simulink model "linefault"  (Simulink 8.5)
settings: Solver=ode15s  SolverMode=SingleTasking  StartTime=0.0  StopTime=0.1  RelTol=1e-3  AbsTol=1e-6
libraries: powerlib x43, powerlib_extras x1
settings Model: Creator=Dr. Lotfifard  LastModifiedBy=PC  ExtModeTrigMode=oneshot  ExtModeArmWhenConnect=off
settings SolverCC: ZeroCrossAlgorithm=Adaptive
settings DataIOCC: LimitDataPoints=off
settings OptimizationCC: BlockReduction=off  BooleanDataType=off
settings DebuggingCC: SaveWithParameterizedLinksMsg=none  SignalResolutionControl=TryResolveAllWithWarning  MultiTaskDSMMsg=warning  MultiTaskCondExecSysMsg=none  FcnCallInpInsideContextMsg=UseLocalSettings
settings HardwareCC: TargetUnknown=on

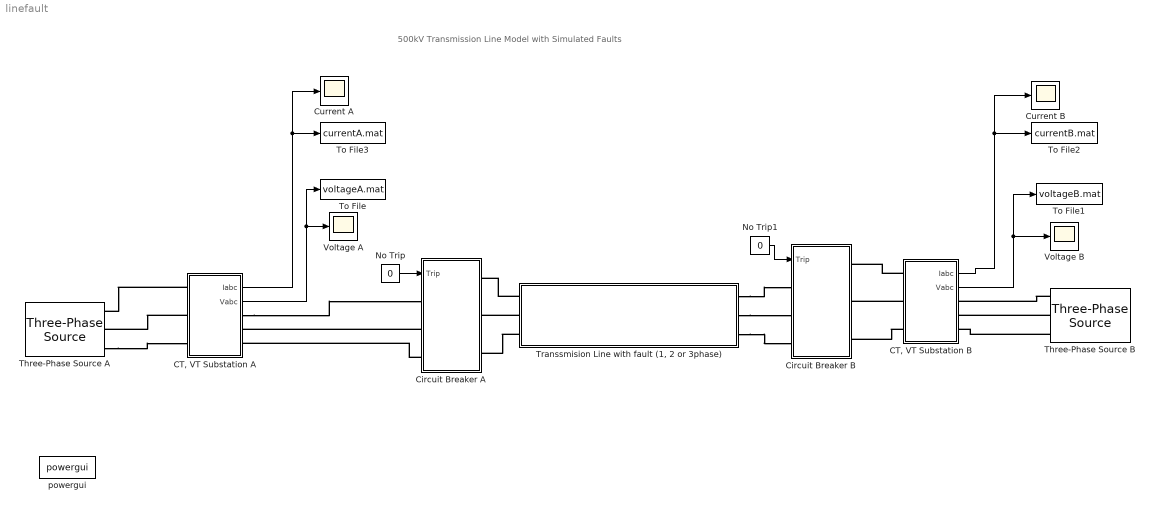
== system linefault ==
  note: 500kV Transmission Line Model with Simulated Faults
  "CT, VT Substation A" : Subsystem  mask{VT=1, CT=1}
      mask prompts: VT "VT ratio"; CT "CT ratio"
  "CT, VT Substation B" : Subsystem  mask{VT=1, CT=1}
      mask prompts: VT "VT ratio"; CT "CT ratio"
  Circuit Breaker A : Subsystem
  Circuit Breaker B : Subsystem
  Current A : Scope
      settings: TickLabels=on  YMin=-8000  YMax=9000
  Current B : Scope
      settings: TickLabels=on
  No Trip : Constant  Value=0
  No Trip1 : Constant  Value=0
  Three-Phase Source A : powerlib/Electrical Sources/Three-Phase Source  Voltage=500000/sqrt(3)*sqrt(2)  PhaseAngle=0  Frequency=60  InternalConnection=Yg  SpecifyImpedance=off  Resistance=0.724  Inductance=19.2e-3  ShortCircuitLevel=100e6  BaseVoltage=25e3  XRratio=7  BusType=swing  Pref=0  Qref=0  Qmin=-inf  Qmax=inf
  Three-Phase Source B : powerlib/Electrical Sources/Three-Phase Source  Voltage=1.05*500000/sqrt(3)*sqrt(2)  PhaseAngle=10  Frequency=60  InternalConnection=Yg  SpecifyImpedance=off  Resistance=0.724  Inductance=19.2e-3  ShortCircuitLevel=100e6  BaseVoltage=25e3  XRratio=7  BusType=swing  Pref=0  Qref=0  Qmin=-inf  Qmax=inf
  To File : ToFile  Filename=voltageA.mat
  To File1 : ToFile  Filename=voltageB.mat
  To File2 : ToFile  Filename=currentB.mat
  To File3 : ToFile  Filename=currentA.mat
  "Transsmision Line with fault (1, 2 or 3phase)" : Subsystem  mask(Teansmission line with fault){ff=60, rr=[0.025485 0.57504], ll=[1.5760e-3 4.5291e-3], cc=[19.1e-9 11.2e-9], length=200, faultLocation=0.1, faultType='A-B', faultR=1, faultTime=[0.034 0.1 0.2 0.5 1]}
      mask prompts: ff "Frequency used for R L C specification (Hz)"; rr "Resistance per unit length (Ohm/km) [R1 R0]"; ll "Inductance per unit length (H/km) [L1 L0]"; cc "Capacitance per unit length (F/km) [C1 C0]"; length "Line length (km)"; faultLocation "Fault location (p.u.) <0,1>"; faultType "Fault Type"; faultR "Fault Resistance per Phase (Ohm)"; faultTime "Fault time sequence (s) [C O C O C]"
      mask TypeOptions faultType: 'A-G' | 'A-B' | 'A-B-G' | 'A-B-C' | 'A-B-C-G'
  Voltage A : Scope
      settings: TickLabels=on
  Voltage B : Scope
      settings: TickLabels=on
  powergui : powerlib/powergui  SimulationMode=Continuous  SolverType=Tustin/Backward Euler (TBE)  SampleTime=0  frequency=60  SPID=off  DisableSnubberDevices=off  DisableRonSwitches=off  DisableVfSwitches=off  SwTol=0  DisplayEquations=off  Interpol=off  methode=off  Ts=0  FunctionMessages=off  echomessages=off  HookPort=off  EnableUseOfTLC=off  x0status=blocks  frequencyindice=60  Pbase=100e6  ErrMax=1e-4  Iterations=50  UnitsV=kV  UnitsW=MW  buscounter=0  RestoreLinks=warning  ResistiveCurrentMeasurement=off  Frange=[0:2:500]  Ylog=off  Xlog=on  ShowGrid=off  save=off  variable=ZData  structure=0  ZoomFFT=on  StartTime=0.0  cycles=1  DisplayStyle=1  fundamental=60  FreqAxis=off  MaxFrequency=1000  frequencyindicesteady=1  RmsSteady=1  display=off
  wires:
  No Trip/1 -> Circuit Breaker A/1(Trip)
  "CT, VT Substation A"/2(Vabc) -> Voltage A/1, To File/1
  No Trip1/1 -> Circuit Breaker B/1(Trip)
  "CT, VT Substation B"/1(Iabc) -> To File2/1, Current B/1
  "CT, VT Substation B"/2(Vabc) -> Voltage B/1, To File1/1
  "CT, VT Substation A"/1(Iabc) -> To File3/1, Current A/1
  connections:
  "CT, VT Substation A"/LConn1 -- Three-Phase Source A/RConn1
  Circuit Breaker A/LConn3 -- "CT, VT Substation A"/RConn3
  "CT, VT Substation B"/LConn2 -- Circuit Breaker B/RConn2
  "CT, VT Substation B"/LConn1 -- Circuit Breaker B/RConn1
  "CT, VT Substation B"/LConn3 -- Circuit Breaker B/RConn3
  Three-Phase Source B/RConn2 -- "CT, VT Substation B"/RConn2
  Three-Phase Source B/RConn1 -- "CT, VT Substation B"/RConn1
  Three-Phase Source B/RConn3 -- "CT, VT Substation B"/RConn3
  "Transsmision Line with fault (1, 2 or 3phase)"/LConn3 -- Circuit Breaker A/RConn3
  "Transsmision Line with fault (1, 2 or 3phase)"/LConn2 -- Circuit Breaker A/RConn2
  "Transsmision Line with fault (1, 2 or 3phase)"/LConn1 -- Circuit Breaker A/RConn1
  "Transsmision Line with fault (1, 2 or 3phase)"/RConn1 -- Circuit Breaker B/LConn1
  "Transsmision Line with fault (1, 2 or 3phase)"/RConn2 -- Circuit Breaker B/LConn2
  "Transsmision Line with fault (1, 2 or 3phase)"/RConn3 -- Circuit Breaker B/LConn3
  Three-Phase Source A/RConn3 -- "CT, VT Substation A"/LConn3
  "CT, VT Substation A"/LConn2 -- Three-Phase Source A/RConn2
  "CT, VT Substation A"/RConn1 -- Circuit Breaker A/LConn1
  Circuit Breaker A/LConn2 -- "CT, VT Substation A"/RConn2

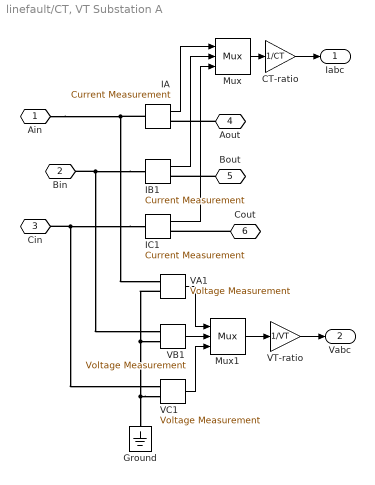
== system linefault/CT, VT Substation A ==
  CT-ratio : Gain  Gain=1/CT  SaturateOnIntegerOverflow=on  OutDataTypeStr=Inherit: Same as input  ParamDataTypeStr=Inherit: Same as input
  Ground : powerlib/Elements/Ground  LConnTagsString=a
  IA : powerlib/Measurements/Current Measurement  PhasorSimulation=off  OutputType=Complex  PSBequivalent=0
  IB1 : powerlib/Measurements/Current Measurement  PhasorSimulation=off  OutputType=Complex  PSBequivalent=0
  IC1 : powerlib/Measurements/Current Measurement  PhasorSimulation=off  OutputType=Complex  PSBequivalent=0
  Mux : Mux  Inputs=3
  Mux1 : Mux  Inputs=3
  VA1 : powerlib/Measurements/Voltage Measurement  PhasorSimulation=off  OutputType=Complex  PSBequivalent=0
  VB1 : powerlib/Measurements/Voltage Measurement  PhasorSimulation=off  OutputType=Complex  PSBequivalent=0
  VC1 : powerlib/Measurements/Voltage Measurement  PhasorSimulation=off  OutputType=Complex  PSBequivalent=0
  VT-ratio : Gain  Gain=1/VT  SaturateOnIntegerOverflow=on  OutDataTypeStr=Inherit: Same as input  ParamDataTypeStr=Inherit: Same as input
  Ain : PMIOPort  Port=1  Side=Left
  Bin : PMIOPort  Port=2  Side=Left
  Cin : PMIOPort  Port=3  Side=Left
  Aout : PMIOPort  Port=4  Side=Right
  Bout : PMIOPort  Port=5  Side=Right
  Cout : PMIOPort  Port=6  Side=Right
  Iabc : Outport
  Vabc : Outport  Port=2
  wires:
  Mux/1 -> CT-ratio/1
  Mux1/1 -> VT-ratio/1
  IA/1 -> Mux/1
  IB1/1 -> Mux/2
  IC1/1 -> Mux/3
  VC1/1 -> Mux1/3
  VB1/1 -> Mux1/2
  VA1/1 -> Mux1/1
  CT-ratio/1 -> Iabc/1
  VT-ratio/1 -> Vabc/1
  connections:
  VC1/LConn2 -- Ground/LConn1 -- VB1/LConn2 -- VA1/LConn2
  Ain/RConn1 -- IA/LConn1 -- VA1/LConn1
  IB1/LConn1 -- Bin/RConn1 -- VB1/LConn1
  IC1/LConn1 -- Cin/RConn1 -- VC1/LConn1
  Cout/RConn1 -- IC1/RConn1
  Aout/RConn1 -- IA/RConn1
  Bout/RConn1 -- IB1/RConn1

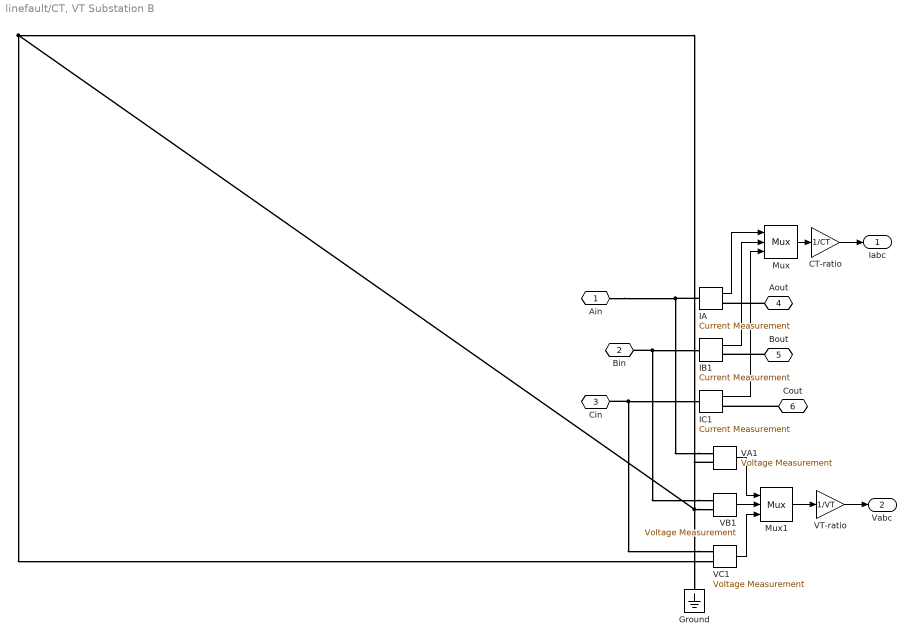
== system linefault/CT, VT Substation B ==
  CT-ratio : Gain  Gain=1/CT  SaturateOnIntegerOverflow=on  OutDataTypeStr=Inherit: Same as input  ParamDataTypeStr=Inherit: Same as input
  Ground : powerlib/Elements/Ground  LConnTagsString=a
  IA : powerlib/Measurements/Current Measurement  PhasorSimulation=off  OutputType=Complex  PSBequivalent=0
  IB1 : powerlib/Measurements/Current Measurement  PhasorSimulation=off  OutputType=Complex  PSBequivalent=0
  IC1 : powerlib/Measurements/Current Measurement  PhasorSimulation=off  OutputType=Complex  PSBequivalent=0
  Mux : Mux  Inputs=3
  Mux1 : Mux  Inputs=3
  VA1 : powerlib/Measurements/Voltage Measurement  PhasorSimulation=off  OutputType=Complex  PSBequivalent=0
  VB1 : powerlib/Measurements/Voltage Measurement  PhasorSimulation=off  OutputType=Complex  PSBequivalent=0
  VC1 : powerlib/Measurements/Voltage Measurement  PhasorSimulation=off  OutputType=Complex  PSBequivalent=0
  VT-ratio : Gain  Gain=1/VT  SaturateOnIntegerOverflow=on  OutDataTypeStr=Inherit: Same as input  ParamDataTypeStr=Inherit: Same as input
  Ain : PMIOPort  Port=1  Side=Left
  Bin : PMIOPort  Port=2  Side=Left
  Cin : PMIOPort  Port=3  Side=Left
  Aout : PMIOPort  Port=4  Side=Right
  Bout : PMIOPort  Port=5  Side=Right
  Cout : PMIOPort  Port=6  Side=Right
  Iabc : Outport
  Vabc : Outport  Port=2
  wires:
  Mux/1 -> CT-ratio/1
  Mux1/1 -> VT-ratio/1
  IA/1 -> Mux/1
  IB1/1 -> Mux/2
  IC1/1 -> Mux/3
  VC1/1 -> Mux1/3
  VB1/1 -> Mux1/2
  VA1/1 -> Mux1/1
  CT-ratio/1 -> Iabc/1
  VT-ratio/1 -> Vabc/1
  connections:
  VB1/LConn2 -- VA1/LConn2 -- VC1/LConn2 -- Ground/LConn1
  VA1/LConn1 -- Ain/RConn1 -- IA/LConn1
  VB1/LConn1 -- IB1/LConn1 -- Bin/RConn1
  VC1/LConn1 -- IC1/LConn1 -- Cin/RConn1
  Cout/RConn1 -- IC1/RConn1
  Aout/RConn1 -- IA/RConn1
  Bout/RConn1 -- IB1/RConn1

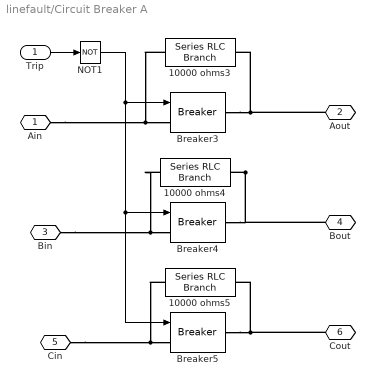
== system linefault/Circuit Breaker A ==
  Trip : Inport
  10000 ohms3 : powerlib/Elements/Series RLC Branch  LConnTagsString=__new0  RConnTagsString=__new0  BranchType=R  Resistance=10000  Inductance=1e-3  SetiL0=off  InitialCurrent=0  Capacitance=1e-6  Setx0=off  InitialVoltage=0  Measurements=None
  10000 ohms4 : powerlib/Elements/Series RLC Branch  LConnTagsString=__new0  RConnTagsString=__new0  BranchType=R  Resistance=10000  Inductance=1e-3  SetiL0=off  InitialCurrent=0  Capacitance=1e-6  Setx0=off  InitialVoltage=0  Measurements=None
  10000 ohms5 : powerlib/Elements/Series RLC Branch  LConnTagsString=__new0  RConnTagsString=__new0  BranchType=R  Resistance=10000  Inductance=1e-3  SetiL0=off  InitialCurrent=0  Capacitance=1e-6  Setx0=off  InitialVoltage=0  Measurements=None
  Breaker3 : powerlib/Elements/Breaker  InitialState=0  SwitchingTimes="[ 1/60  5/60 ]"  External=on  BreakerResistance=0.01  SnubberResistance=1e6  SnubberCapacitance=inf  Measurements=None  MoreParameters=off  NoBreakLoop=off
  Breaker4 : powerlib/Elements/Breaker  InitialState=0  SwitchingTimes="[ 1/60  5/60 ]"  External=on  BreakerResistance=0.01  SnubberResistance=1e6  SnubberCapacitance=inf  Measurements=None  MoreParameters=off  NoBreakLoop=off
  Breaker5 : powerlib/Elements/Breaker  InitialState=0  SwitchingTimes="[ 1/60  5/60 ]"  External=on  BreakerResistance=0.01  SnubberResistance=1e6  SnubberCapacitance=inf  Measurements=None  MoreParameters=off  NoBreakLoop=off
  NOT1 : Logic  Operator=NOT  Inputs=1
  Ain : PMIOPort  Port=1  Side=Left
  Aout : PMIOPort  Port=2  Side=Right
  Bin : PMIOPort  Port=3  Side=Right
  Bout : PMIOPort  Port=4  Side=Left
  Cin : PMIOPort  Port=5  Side=Left
  Cout : PMIOPort  Port=6  Side=Right
  wires:
  Trip/1 -> NOT1/1
  NOT1/1 -> Breaker3/1, Breaker4/1, Breaker5/1
  connections:
  10000 ohms3/LConn1 -- Ain/RConn1 -- Breaker3/LConn1
  Aout/RConn1 -- 10000 ohms3/RConn1 -- Breaker3/RConn1
  10000 ohms4/LConn1 -- Bin/RConn1 -- Breaker4/LConn1
  10000 ohms4/RConn1 -- Bout/RConn1 -- Breaker4/RConn1
  10000 ohms5/LConn1 -- Cin/RConn1 -- Breaker5/LConn1
  Cout/RConn1 -- 10000 ohms5/RConn1 -- Breaker5/RConn1

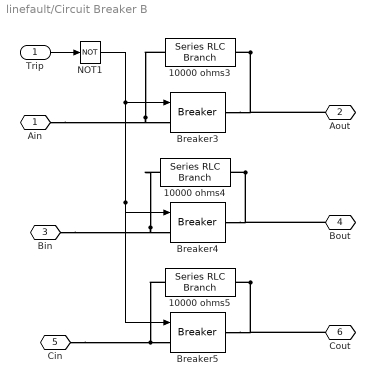
== system linefault/Circuit Breaker B ==
  Trip : Inport
  10000 ohms3 : powerlib/Elements/Series RLC Branch  LConnTagsString=__new0  RConnTagsString=__new0  BranchType=R  Resistance=10000  Inductance=1e-3  SetiL0=off  InitialCurrent=0  Capacitance=1e-6  Setx0=off  InitialVoltage=0  Measurements=None
  10000 ohms4 : powerlib/Elements/Series RLC Branch  LConnTagsString=__new0  RConnTagsString=__new0  BranchType=R  Resistance=10000  Inductance=1e-3  SetiL0=off  InitialCurrent=0  Capacitance=1e-6  Setx0=off  InitialVoltage=0  Measurements=None
  10000 ohms5 : powerlib/Elements/Series RLC Branch  LConnTagsString=__new0  RConnTagsString=__new0  BranchType=R  Resistance=10000  Inductance=1e-3  SetiL0=off  InitialCurrent=0  Capacitance=1e-6  Setx0=off  InitialVoltage=0  Measurements=None
  Breaker3 : powerlib/Elements/Breaker  InitialState=0  SwitchingTimes="[ 1/60  5/60 ]"  External=on  BreakerResistance=0.01  SnubberResistance=1e6  SnubberCapacitance=inf  Measurements=None  MoreParameters=off  NoBreakLoop=off
  Breaker4 : powerlib/Elements/Breaker  InitialState=0  SwitchingTimes="[ 1/60  5/60 ]"  External=on  BreakerResistance=0.01  SnubberResistance=1e6  SnubberCapacitance=inf  Measurements=None  MoreParameters=off  NoBreakLoop=off
  Breaker5 : powerlib/Elements/Breaker  InitialState=0  SwitchingTimes="[ 1/60  5/60 ]"  External=on  BreakerResistance=0.01  SnubberResistance=1e6  SnubberCapacitance=inf  Measurements=None  MoreParameters=off  NoBreakLoop=off
  NOT1 : Logic  Operator=NOT  Inputs=1
  Ain : PMIOPort  Port=1  Side=Left
  Aout : PMIOPort  Port=2  Side=Right
  Bin : PMIOPort  Port=3  Side=Right
  Bout : PMIOPort  Port=4  Side=Left
  Cin : PMIOPort  Port=5  Side=Left
  Cout : PMIOPort  Port=6  Side=Right
  wires:
  Trip/1 -> NOT1/1
  NOT1/1 -> Breaker3/1, Breaker4/1, Breaker5/1
  connections:
  10000 ohms3/LConn1 -- Ain/RConn1 -- Breaker3/LConn1
  10000 ohms3/RConn1 -- Aout/RConn1 -- Breaker3/RConn1
  10000 ohms4/LConn1 -- Bin/RConn1 -- Breaker4/LConn1
  10000 ohms4/RConn1 -- Bout/RConn1 -- Breaker4/RConn1
  10000 ohms5/LConn1 -- Cin/RConn1 -- Breaker5/LConn1
  10000 ohms5/RConn1 -- Cout/RConn1 -- Breaker5/RConn1

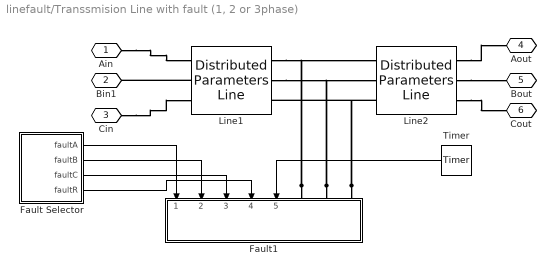
== system linefault/Transsmision Line with fault (1, 2 or 3phase) ==
  Fault Selector : Subsystem
  Fault1 : Subsystem
  Line1 : powerlib/Elements/Distributed Parameters Line  Phases=3  Frequency=ff  Resistance=rr  Inductance=ll  Capacitance=cc  Length=length*(faultLocation+0.0005)  x1=[0 1.53266796670346e-009 -40255.985134743 -39683.0380465592;2.86312968195295e-005 1.53189939694959e-009 -39825.3198862797 -40115.2308198371;5.7262593639059e-005 1.53095235510765e-009 -39390.0148370482 -40542.7500166237;8.58938904585885e-005 1.52982695151157e-009 -38950.120701737 -40965.5458293116;0.000114525187278118 1.52852331727516e-009 -38505.688729681 -41383.5690005856;0.000143156484097647 1.52704160427675e-009 -38056.77069889 -41796.7708291612]  x2=[0 1.55925131848491e-009 -40620.0878760363 -39910.0233219334;2.86312968195295e-005 1.55881129165316e-009 -40186.9514443784 -40346.1328285791;5.7262593639059e-005 1.55818965739555e-009 -39749.1330805045 -40777.5418577741;8.58938904585885e-005 1.55738648813482e-009 -39306.6837919141 -41204.2001487306;0.000114525187278118 1.55640187744325e-009 -38859.6551256268 -41626.0579941401;0.000143156484097647 1.55523594003171e-009 -38408.0991621773 -42043.0662459641]  x3=[0 2.01885457122014e-012 -163.089263474603 -105.450555147554;2.86312968195295e-005 2.03239610658583e-012 -161.941578955542 -107.204722130146;5.7262593639059e-005 2.04570086009907e-012 -160.775027628515 -108.946399356132;8.58938904585885e-005 2.05876728170564e-012 -159.589745401176 -110.675383913513;0.000114525187278118 2.07159384911787e-012 -158.385870363398 -112.391474369031;0.000143156484097647 2.08417906799204e-012 -157.163542771187 -114.094470791643]  x4=[0 2.64131154335596e-012 -123.841881809461 -165.416317671308;2.86312968195295e-005 2.63470626197041e-012 -122.049240966749 -166.743373545949;5.7262593639059e-005 2.62779402731559e-012 -120.242380924704 -168.051003185349;8.58938904585885e-005 2.62057564469306e-012 -118.42151218937 -169.339054245695;0.000114525187278118 2.61305195507176e-012 -116.58684689886 -170.607376664157;0.000143156484097647 2.60522383499005e-012 -114.738598798635 -171.855822676363]  x5=0.000143156484097647  V1=[1.853e-09 5.653e+04 5.653e+04;377 377 377;2.194 -0.7926 -2.363]  V2=[1.919e-09 5.695e+04 5.695e+04;377 377 377;2.197 -0.7942 -2.365]  I1=[3.629e-12 194.2 194.2;377 377 377;1.661 -0.9968 -2.568]  I2=[2.446e-12 206.6 206.6;377 377 377;2.735 -0.6426 -2.213]  nHarmo=1  Measurements=None
  Line2 : powerlib/Elements/Distributed Parameters Line  Phases=3  Frequency=ff  Resistance=rr  Inductance=ll  Capacitance=cc  Length=length*(1-faultLocation-0.0005)  x1=[0 1.43137261755031e-009 -51373.762200412 -24567.0115803634;0.000256257228747928 1.48443013216827e-009 -48764.5687185778 -29407.7938360784;0.000512514457495856 1.52364444798437e-009 -45700.6164679546 -33974.3308258324;0.000768771686243784 1.54864986805002e-009 -42210.4786357914 -38224.0368610064;0.00102502891499171 1.55921320186769e-009 -38326.7028447818 -42117.2808911256;0.00128128614373964 1.55523594003171e-009 -34085.5076270153 -45617.7560871077]  x2=[0 1.5552865834267e-009 -50810.114798948 -24266.9121672487;0.000256257228747928 1.62275226289842e-009 -48232.4960307204 -29054.7262706394;0.000512514457495856 1.67508480697045e-009 -45205.080389744 -33571.5876742822;0.000768771686243784 1.71179618336988e-009 -41756.1003375311 -37775.3739441089;0.00102502891499171 1.73254403655516e-009 -37917.719675861 -41626.8822589206;0.00128128614373964 1.73713488038629e-009 -33725.7336000921 -45090.195000142]  x3=[0 1.4523601474402e-012 -189.596238125285 -56.3258357388615;0.000256257228747928 1.62464711268222e-012 -183.279195992341 -74.3509892290754;0.000512514457495856 1.78178327191703e-012 -175.252965739737 -91.6827752763165;0.000768771686243784 1.92230323647857e-012 -165.592396764968 -108.159564609767;0.00102502891499171 2.04489657365404e-012 -154.387579651591 -123.627701314326;0.00128128614373964 2.14842002725272e-012 -141.743006020653 -137.942935763923]  x4=[0 2.19293673092143e-012 -193.598935066748 -45.2078125315412;0.000256257228747928 2.29222269793401e-012 -188.335634767859 -63.6708932672806;0.000512514457495856 2.37013231733818e-012 -181.315992033535 -81.540204842525;0.000768771686243784 2.42593903533621e-012 -172.605469230635 -98.64910523942;0.00102502891499171 2.45912242090544e-012 -162.285297193952 -114.838043729142;0.00128128614373964 2.46937301912888e-012 -150.451717700097 -129.956048777869]  x5=0.00128128614373964  V1=[1.919e-09 5.695e+04 5.695e+04;377 377 377;1.768 -1.125 -2.696]  V2=[2.119e-09 5.631e+04 5.631e+04;377 377 377;1.69 -1.125 -2.696]  I1=[2.695e-12 197.8 197.8;377 377 377;1.234 -1.282 -2.853]  I2=[3.178e-12 198.8 198.8;377 377 377;1.693 -1.341 -2.912]  nHarmo=1  Measurements=None
  Timer : powerlib_extras/Control  Blocks/Timer  t=[0 faultTime]  e=[0 1 0 1 0 1]
  Ain : PMIOPort  Port=1  Side=Left
  Bin1 : PMIOPort  Port=2  Side=Left
  Cin : PMIOPort  Port=3  Side=Left
  Aout : PMIOPort  Port=4  Side=Right
  Bout : PMIOPort  Port=5  Side=Right
  Cout : PMIOPort  Port=6  Side=Right
  wires:
  Timer/1 -> Fault1/5(Tfault)
  Fault Selector/1(faultA) -> Fault1/1(faultA)
  Fault Selector/2(faultB) -> Fault1/2(faultB)
  Fault Selector/3(faultC) -> Fault1/3(faultC)
  Fault Selector/4(faultR) -> Fault1/4(faultG)
  connections:
  Fault1/LConn1 -- Line2/LConn1 -- Line1/RConn1
  Fault1/LConn2 -- Line1/RConn2 -- Line2/LConn2
  Fault1/LConn3 -- Line2/LConn3 -- Line1/RConn3
  Cin/RConn1 -- Line1/LConn3
  Line1/LConn2 -- Bin1/RConn1
  Line2/RConn3 -- Cout/RConn1
  Ain/RConn1 -- Line1/LConn1
  Line2/RConn2 -- Bout/RConn1
  Line2/RConn1 -- Aout/RConn1

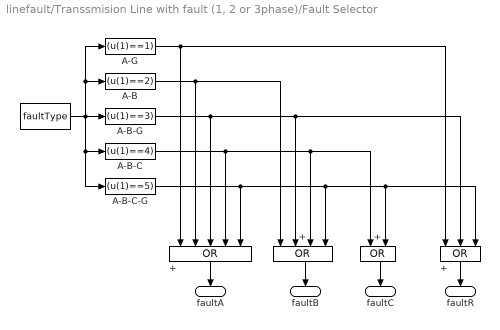
== system linefault/Transsmision Line with fault (1, 2 or 3phase)/Fault Selector ==
  "  " : Constant  Value=faultType
  "  +" : Logic  Operator=OR
  " +" : Logic  Operator=OR  Inputs=4
  + : Logic  Operator=OR  Inputs=5
  "+ " : Logic  Operator=OR  Inputs=3
  A-B : Fcn  Expr=(u(1)==2)
  A-B-C : Fcn  Expr=(u(1)==4)
  A-B-C-G : Fcn  Expr=(u(1)==5)
  A-B-G : Fcn  Expr=(u(1)==3)
  A-G : Fcn  Expr=(u(1)==1)
  faultA : Outport  InitialOutput=0
  faultB : Outport  Port=2  InitialOutput=0
  faultC : Outport  Port=3  InitialOutput=0
  faultR : Outport  Port=4  InitialOutput=0
  wires:
  "  "/1 -> A-B-G/1, A-G/1, A-B/1, A-B-C-G/1, A-B-C/1
  +/1 -> faultA/1
  " +"/1 -> faultB/1
  "  +"/1 -> faultC/1
  "+ "/1 -> faultR/1
  A-B/1 -> +/2, " +"/1
  A-B-G/1 -> +/3, " +"/2, "+ "/2
  A-B-C/1 -> +/4, " +"/3, "  +"/1
  A-B-C-G/1 -> +/5, " +"/4, "  +"/2, "+ "/3
  A-G/1 -> +/1, "+ "/1

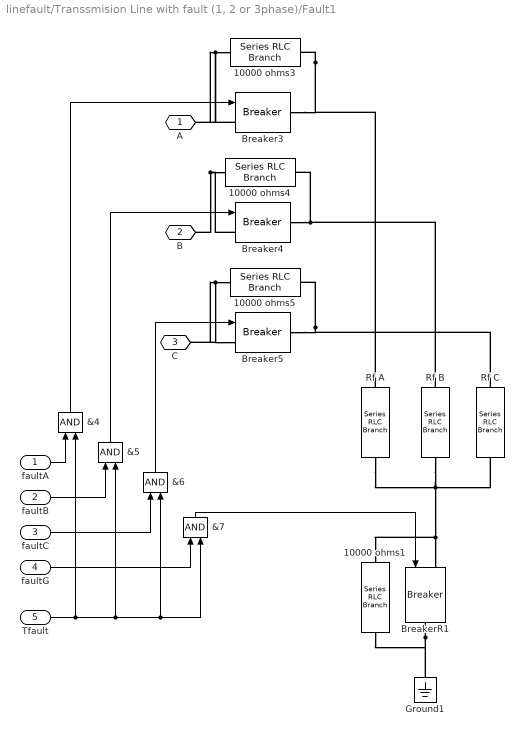
== system linefault/Transsmision Line with fault (1, 2 or 3phase)/Fault1 ==
  faultA : Inport
  faultB : Inport  Port=2
  faultC : Inport  Port=3
  faultG : Inport  Port=4
  Tfault : Inport  Port=5
  &{4..7} (4 alike) : Logic
  10000 ohms{1,3..5} (4 alike) : powerlib/Elements/Series RLC Branch  LConnTagsString=__new0  RConnTagsString=__new0  BranchType=R  Resistance=10000  Inductance=1e-3  SetiL0=off  InitialCurrent=0  Capacitance=1e-6  Setx0=off  InitialVoltage=0  Measurements=None
  Breaker3 : powerlib/Elements/Breaker  InitialState=0  SwitchingTimes="[ 1/60  5/60 ]"  External=on  BreakerResistance=0.01  SnubberResistance=1e6  SnubberCapacitance=inf  Measurements=None  MoreParameters=off  NoBreakLoop=off
  Breaker4 : powerlib/Elements/Breaker  InitialState=0  SwitchingTimes="[ 1/60  5/60 ]"  External=on  BreakerResistance=0.01  SnubberResistance=1e6  SnubberCapacitance=inf  Measurements=None  MoreParameters=off  NoBreakLoop=off
  Breaker5 : powerlib/Elements/Breaker  InitialState=0  SwitchingTimes="[ 1/60  5/60 ]"  External=on  BreakerResistance=0.01  SnubberResistance=1e6  SnubberCapacitance=inf  Measurements=None  MoreParameters=off  NoBreakLoop=off
  BreakerR1 : powerlib/Elements/Breaker  InitialState=0  SwitchingTimes="[ 1/60  5/60 ]"  External=on  BreakerResistance=0.01  SnubberResistance=1e6  SnubberCapacitance=inf  Measurements=None  MoreParameters=off  NoBreakLoop=off
  Ground1 : powerlib/Elements/Ground  LConnTagsString=a
  Rf A : powerlib/Elements/Series RLC Branch  LConnTagsString=__new0  RConnTagsString=__new0  BranchType=R  Resistance=faultR  Inductance=0  SetiL0=off  InitialCurrent=0  Capacitance=1e-6  Setx0=off  InitialVoltage=0  Measurements=None
  Rf B : powerlib/Elements/Series RLC Branch  LConnTagsString=__new0  RConnTagsString=__new0  BranchType=R  Resistance=faultR  Inductance=0  SetiL0=off  InitialCurrent=0  Capacitance=1e-6  Setx0=off  InitialVoltage=0  Measurements=None
  Rf C : powerlib/Elements/Series RLC Branch  LConnTagsString=__new0  RConnTagsString=__new0  BranchType=R  Resistance=faultR  Inductance=0  SetiL0=off  InitialCurrent=0  Capacitance=1e-6  Setx0=off  InitialVoltage=0  Measurements=None
  A : PMIOPort  Port=1  Side=Left
  B : PMIOPort  Port=2  Side=Left
  C : PMIOPort  Port=3  Side=Left
  wires:
  &6/1 -> Breaker5/1
  &5/1 -> Breaker4/1
  Tfault/1 -> &7/2, &6/2, &5/2, &4/2
  &7/1 -> BreakerR1/1
  faultG/1 -> &7/1
  faultC/1 -> &6/1
  faultB/1 -> &5/1
  faultA/1 -> &4/1
  &4/1 -> Breaker3/1
  connections:
  Rf B/RConn1 -- Rf C/RConn1 -- BreakerR1/LConn1 -- 10000 ohms1/LConn1 -- Rf A/RConn1
  BreakerR1/RConn1 -- 10000 ohms1/RConn1 -- Ground1/LConn1
  10000 ohms3/LConn1 -- A/RConn1 -- Breaker3/LConn1
  Rf A/LConn1 -- 10000 ohms3/RConn1 -- Breaker3/RConn1
  10000 ohms4/LConn1 -- B/RConn1 -- Breaker4/LConn1
  Rf B/LConn1 -- 10000 ohms4/RConn1 -- Breaker4/RConn1
  10000 ohms5/LConn1 -- C/RConn1 -- Breaker5/LConn1
  Rf C/LConn1 -- 10000 ohms5/RConn1 -- Breaker5/RConn1
